simulink model "fitzhugh_relay_gain_added"  (R2015a)
settings: Solver=ode45  StartTime=0.0  StopTime=1  RelTol=1e-3
settings Model: Creator=ra428  LastModifiedBy=ra428

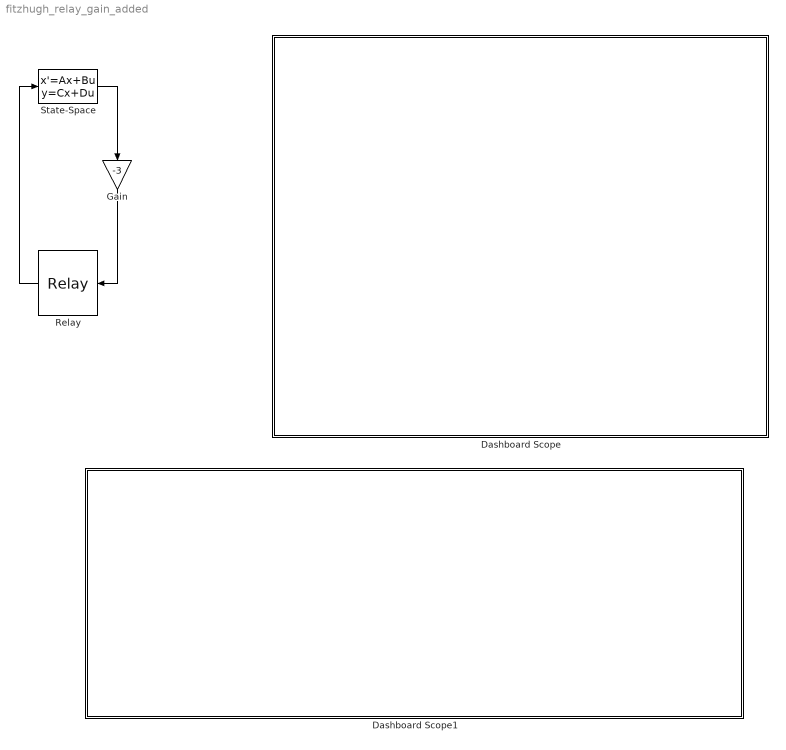
== system fitzhugh_relay_gain_added ==
  Dashboard Scope : Subsystem  DialogController=hmiCreateDDGDialog  IsWebBlock=on  mask(MathWorksWebBlock){webBlockId=b8900825-483f-4ab5-a2e3-572b6d00bd2c, webBlockType=sdiscope, ShowInitialText=on, HMISrcModelName=untitled}
      mask prompts: webBlockId "WebBlock Id"; webBlockType "WebBlock Type"; HMISrcModelName "Source Model"
      mask Help: helpview([docroot '/mapfiles/simulink.map'], 'hmi_scope')
      mask Display:
      | if strcmp(get_param(bdroot(gcb),'BlockDiagramType'), 'library')
      |     image([(matlabroot) '/toolbox/simulink/hmi/icons/DashboardScope.png']);
      | end
  Dashboard Scope1 : Subsystem  DialogController=hmiCreateDDGDialog  IsWebBlock=on  mask(MathWorksWebBlock){webBlockId=ba074387-6b97-4300-9462-7d768d333b01, webBlockType=sdiscope, ShowInitialText=on, HMISrcModelName=untitled}
      mask prompts: webBlockId "WebBlock Id"; webBlockType "WebBlock Type"; HMISrcModelName "Source Model"
      mask Help: helpview([docroot '/mapfiles/simulink.map'], 'hmi_scope')
      mask Display:
      | if strcmp(get_param(bdroot(gcb),'BlockDiagramType'), 'library')
      |     image([(matlabroot) '/toolbox/simulink/hmi/icons/DashboardScope.png']);
      | end
  Gain : Gain  Gain=-3
  Relay : Relay  OnSwitchValue=0.663  OffSwitchValue=0.4758  OnOutputValue=0.505  OffOutputValue=-0.2876
  State-Space : StateSpace  A=-0.5  D=0  X0=-0.2
  wires:
  Gain/1 -> Relay/1
  Relay/1 -> State-Space/1
  State-Space/1 -> Gain/1

== system fitzhugh_relay_gain_added/Dashboard Scope ==

== system fitzhugh_relay_gain_added/Dashboard Scope1 ==
